simulink model "hoppingControl"  (R2018b)
settings: Solver=FixedStepAuto  StartTime=0.0  StopTime=inf  RelTol=1e-3  EnableMultiTasking=on
libraries: dspstat3 x19, cm_custom x9, raspberrypilib x8, simulink_extras x3, peGeneralControl x3, can_bus_multi x2, simulink x1, embdlinuxlib x1
(part 3 of 3)

== matlab function hoppingControl/Kinematics/MATLAB Function6 ==
  data: theta input; pos output; D input; d input; r input; check output
function [pos, check] = forward_kinematics(theta,D,d,r)
s1 = sin(theta(1)); s2 = sin(theta(2)); s3=sin(theta(3));
c1 = cos(theta(1)); c2 = cos(theta(2)); c3=cos(theta(3));

pos = zeros([3,1]);
knee = zeros([3,3]);
pos(1) =(3^(1/2)*(3*r^3 + D^3*c1*c2^2 + D^3*c2^2*c3 + 2*D*r^2*c1 + 3*D*r^2*c2 + 4*D*r^2*c3 + 2*D^2*r*c2^2 + D^2*r*c1*c2 + 3*D^2*r*c1*c3 + 3*D^2*r*c2*c3 + D^3*c1*c2*c3))/(2*(3*r^2 + D^2*c1*c2 + D^2*c1*c3 + D^2*c2*c3 + 2*D*r*c1 + 2*D*r*c2 + 2*D*r*c3)) - (3^(1/2)*r)/2 - (3^(1/2)*D*c2)/2 + (3^(1/2)*D*(((2*D*s2 + (((c2*s1 + c3*s1 - c2*s3 - c3*s2)*D^2 - r*(s2 - 2*s1 + s3)*D)*(3*r^3 + D^3*c1*c2^2 + D^3*c2^2*c3 + 6*D*r^2*c1 + 3*D*r^2*c2 + 2*D^2*r*c2^2 + 5*D^2*r*c1*c2 + 3*D^2*r*c1*c3 - D^2*r*c2*c3 + D^3*c1*c2*c3))/(3*r^2 + D^2*c1*c2 + D^2*c1*c3 + D^2*c2*c3 + 2*D*r*c1 + 2*D*r*c2 + 2*D*r*c3)^2 - (D*(3*D*sin(theta(1) + theta(2)) - 3*D*sin(theta(1) + theta(3)) + 6*r*s2 - 6*r*s3 - D*sin(theta(1) - theta(2)) + D*sin(theta(1) - theta(3)) + 2*D*sin(theta(2) - theta(3)))*(3*r^3 + D^3*c1*c2^2 + D^3*c2^2*c3 + 2*D*r^2*c1 + 3*D*r^2*c2 + 4*D*r^2*c3 + 2*D^2*r*c2^2 + D^2*r*c1*c2 + 3*D^2*r*c1*c3 + 3*D^2*r*c2*c3 + D^3*c1*c2*c3))/(2*(3*r^2 + D^2*c1*c2 + D^2*c1*c3 + D^2*c2*c3 + 2*D*r*c1 + 2*D*r*c2 + 2*D*r*c3)^2))^2 - ((4*((c2*s1 + c3*s1 - c2*s3 - c3*s2)*D^2 - r*(s2 - 2*s1 + s3)*D)^2)/(3*r^2 + D^2*c1*c2 + D^2*c1*c3 + D^2*c2*c3 + 2*D*r*c1 + 2*D*r*c2 + 2*D*r*c3)^2 + (D^2*(3*D*sin(theta(1) + theta(2)) - 3*D*sin(theta(1) + theta(3)) + 6*r*s2 - 6*r*s3 - D*sin(theta(1) - theta(2)) + D*sin(theta(1) - theta(3)) + 2*D*sin(theta(2) - theta(3)))^2)/(3*(3*r^2 + D^2*c1*c2 + D^2*c1*c3 + D^2*c2*c3 + 2*D*r*c1 + 2*D*r*c2 + 2*D*r*c3)^2) + 4)*((3*r^3 + D^3*c1*c2^2 + D^3*c2^2*c3 + 6*D*r^2*c1 + 3*D*r^2*c2 + 2*D^2*r*c2^2 + 5*D^2*r*c1*c2 + 3*D^2*r*c1*c3 - D^2*r*c2*c3 + D^3*c1*c2*c3)^2/(4*(3*r^2 + D^2*c1*c2 + D^2*c1*c3 + D^2*c2*c3 + 2*D*r*c1 + 2*D*r*c2 + 2*D*r*c3)^2) - D^2*(c2^2 - 1) - d^2 + (3*(3*r^3 + D^3*c1*c2^2 + D^3*c2^2*c3 + 2*D*r^2*c1 + 3*D*r^2*c2 + 4*D*r^2*c3 + 2*D^2*r*c2^2 + D^2*r*c1*c2 + 3*D^2*r*c1*c3 + 3*D^2*r*c2*c3 + D^3*c1*c2*c3)^2)/(4*(3*r^2 + D^2*c1*c2 + D^2*c1*c3 + D^2*c2*c3 + 2*D*r*c1 + 2*D*r*c2 + 2*D*r*c3)^2)))^(1/2)/2 + D*s2 + (((c2*s1 + c3*s1 - c2*s3 - c3*s2)*D^2 - r*(s2 - 2*s1 + s3)*D)*(3*r^3 + D^3*c1*c2^2 + D^3*c2^2*c3 + 6*D*r^2*c1 + 3*D*r^2*c2 + 2*D^2*r*c2^2 + 5*D^2*r*c1*c2 + 3*D^2*r*c1*c3 - D^2*r*c2*c3 + D^3*c1*c2*c3))/(2*(3*r^2 + D^2*c1*c2 + D^2*c1*c3 + D^2*c2*c3 + 2*D*r*c1 + 2*D*r*c2 + 2*D*r*c3)^2) - (D*(3*D*sin(theta(1) + theta(2)) - 3*D*sin(theta(1) + theta(3)) + 6*r*s2 - 6*r*s3 - D*sin(theta(1) - theta(2)) + D*sin(theta(1) - theta(3)) + 2*D*sin(theta(2) - theta(3)))*(3*r^3 + D^3*c1*c2^2 + D^3*c2^2*c3 + 2*D*r^2*c1 + 3*D*r^2*c2 + 4*D*r^2*c3 + 2*D^2*r*c2^2 + D^2*r*c1*c2 + 3*D^2*r*c1*c3 + 3*D^2*r*c2*c3 + D^3*c1*c2*c3))/(4*(3*r^2 + D^2*c1*c2 + D^2*c1*c3 + D^2*c2*c3 + 2*D*r*c1 + 2*D*r*c2 + 2*D*r*c3)^2))*(3*D*sin(theta(1) + theta(2)) - 3*D*sin(theta(1) + theta(3)) + 6*r*s2 - 6*r*s3 - D*sin(theta(1) - theta(2)) + D*sin(theta(1) - theta(3)) + 2*D*sin(theta(2) - theta(3))))/(6*(((c2*s1 + c3*s1 - c2*s3 - c3*s2)*D^2 - r*(s2 - 2*s1 + s3)*D)^2/(3*r^2 + D^2*c1*c2 + D^2*c1*c3 + D^2*c2*c3 + 2*D*r*c1 + 2*D*r*c2 + 2*D*r*c3)^2 + (D^2*(3*D*sin(theta(1) + theta(2)) - 3*D*sin(theta(1) + theta(3)) + 6*r*s2 - 6*r*s3 - D*sin(theta(1) - theta(2)) + D*sin(theta(1) - theta(3)) + 2*D*sin(theta(2) - theta(3)))^2)/(12*(3*r^2 + D^2*c1*c2 + D^2*c1*c3 + D^2*c2*c3 + 2*D*r*c1 + 2*D*r*c2 + 2*D*r*c3)^2) + 1)*(3*r^2 + D^2*c1*c2 + D^2*c1*c3 + D^2*c2*c3 + 2*D*r*c1 + 2*D*r*c2 + 2*D*r*c3));
pos(2) = (3*r^3 + D^3*c1*c2^2 + D^3*c2^2*c3 + 6*D*r^2*c1 + 3*D*r^2*c2 + 2*D^2*r*c2^2 + 5*D^2*r*c1*c2 + 3*D^2*r*c1*c3 - D^2*r*c2*c3 + D^3*c1*c2*c3)/(2*(3*r^2 + D^2*c1*c2 + D^2*c1*c3 + D^2*c2*c3 + 2*D*r*c1 + 2*D*r*c2 + 2*D*r*c3)) - r/2 - (D*c2)/2 - (((c2*s1 + c3*s1 - c2*s3 - c3*s2)*D^2 - r*(s2 - 2*s1 + s3)*D)*(((2*D*s2 + (((c2*s1 + c3*s1 - c2*s3 - c3*s2)*D^2 - r*(s2 - 2*s1 + s3)*D)*(3*r^3 + D^3*c1*c2^2 + D^3*c2^2*c3 + 6*D*r^2*c1 + 3*D*r^2*c2 + 2*D^2*r*c2^2 + 5*D^2*r*c1*c2 + 3*D^2*r*c1*c3 - D^2*r*c2*c3 + D^3*c1*c2*c3))/(3*r^2 + D^2*c1*c2 + D^2*c1*c3 + D^2*c2*c3 + 2*D*r*c1 + 2*D*r*c2 + 2*D*r*c3)^2 - (D*(3*D*sin(theta(1) + theta(2)) - 3*D*sin(theta(1) + theta(3)) + 6*r*s2 - 6*r*s3 - D*sin(theta(1) - theta(2)) + D*sin(theta(1) - theta(3)) + 2*D*sin(theta(2) - theta(3)))*(3*r^3 + D^3*c1*c2^2 + D^3*c2^2*c3 + 2*D*r^2*c1 + 3*D*r^2*c2 + 4*D*r^2*c3 + 2*D^2*r*c2^2 + D^2*r*c1*c2 + 3*D^2*r*c1*c3 + 3*D^2*r*c2*c3 + D^3*c1*c2*c3))/(2*(3*r^2 + D^2*c1*c2 + D^2*c1*c3 + D^2*c2*c3 + 2*D*r*c1 + 2*D*r*c2 + 2*D*r*c3)^2))^2 - ((4*((c2*s1 + c3*s1 - c2*s3 - c3*s2)*D^2 - r*(s2 - 2*s1 + s3)*D)^2)/(3*r^2 + D^2*c1*c2 + D^2*c1*c3 + D^2*c2*c3 + 2*D*r*c1 + 2*D*r*c2 + 2*D*r*c3)^2 + (D^2*(3*D*sin(theta(1) + theta(2)) - 3*D*sin(theta(1) + theta(3)) + 6*r*s2 - 6*r*s3 - D*sin(theta(1) - theta(2)) + D*sin(theta(1) - theta(3)) + 2*D*sin(theta(2) - theta(3)))^2)/(3*(3*r^2 + D^2*c1*c2 + D^2*c1*c3 + D^2*c2*c3 + 2*D*r*c1 + 2*D*r*c2 + 2*D*r*c3)^2) + 4)*((3*r^3 + D^3*c1*c2^2 + D^3*c2^2*c3 + 6*D*r^2*c1 + 3*D*r^2*c2 + 2*D^2*r*c2^2 + 5*D^2*r*c1*c2 + 3*D^2*r*c1*c3 - D^2*r*c2*c3 + D^3*c1*c2*c3)^2/(4*(3*r^2 + D^2*c1*c2 + D^2*c1*c3 + D^2*c2*c3 + 2*D*r*c1 + 2*D*r*c2 + 2*D*r*c3)^2) - D^2*(c2^2 - 1) - d^2 + (3*(3*r^3 + D^3*c1*c2^2 + D^3*c2^2*c3 + 2*D*r^2*c1 + 3*D*r^2*c2 + 4*D*r^2*c3 + 2*D^2*r*c2^2 + D^2*r*c1*c2 + 3*D^2*r*c1*c3 + 3*D^2*r*c2*c3 + D^3*c1*c2*c3)^2)/(4*(3*r^2 + D^2*c1*c2 + D^2*c1*c3 + D^2*c2*c3 + 2*D*r*c1 + 2*D*r*c2 + 2*D*r*c3)^2)))^(1/2)/2 + D*s2 + (((c2*s1 + c3*s1 - c2*s3 - c3*s2)*D^2 - r*(s2 - 2*s1 + s3)*D)*(3*r^3 + D^3*c1*c2^2 + D^3*c2^2*c3 + 6*D*r^2*c1 + 3*D*r^2*c2 + 2*D^2*r*c2^2 + 5*D^2*r*c1*c2 + 3*D^2*r*c1*c3 - D^2*r*c2*c3 + D^3*c1*c2*c3))/(2*(3*r^2 + D^2*c1*c2 + D^2*c1*c3 + D^2*c2*c3 + 2*D*r*c1 + 2*D*r*c2 + 2*D*r*c3)^2) - (D*(3*D*sin(theta(1) + theta(2)) - 3*D*sin(theta(1) + theta(3)) + 6*r*s2 - 6*r*s3 - D*sin(theta(1) - theta(2)) + D*sin(theta(1) - theta(3)) + 2*D*sin(theta(2) - theta(3)))*(3*r^3 + D^3*c1*c2^2 + D^3*c2^2*c3 + 2*D*r^2*c1 + 3*D*r^2*c2 + 4*D*r^2*c3 + 2*D^2*r*c2^2 + D^2*r*c1*c2 + 3*D^2*r*c1*c3 + 3*D^2*r*c2*c3 + D^3*c1*c2*c3))/(4*(3*r^2 + D^2*c1*c2 + D^2*c1*c3 + D^2*c2*c3 + 2*D*r*c1 + 2*D*r*c2 + 2*D*r*c3)^2)))/((((c2*s1 + c3*s1 - c2*s3 - c3*s2)*D^2 - r*(s2 - 2*s1 + s3)*D)^2/(3*r^2 + D^2*c1*c2 + D^2*c1*c3 + D^2*c2*c3 + 2*D*r*c1 + 2*D*r*c2 + 2*D*r*c3)^2 + (D^2*(3*D*sin(theta(1) + theta(2)) - 3*D*sin(theta(1) + theta(3)) + 6*r*s2 - 6*r*s3 - D*sin(theta(1) - theta(2)) + D*sin(theta(1) - theta(3)) + 2*D*sin(theta(2) - theta(3)))^2)/(12*(3*r^2 + D^2*c1*c2 + D^2*c1*c3 + D^2*c2*c3 + 2*D*r*c1 + 2*D*r*c2 + 2*D*r*c3)^2) + 1)*(3*r^2 + D^2*c1*c2 + D^2*c1*c3 + D^2*c2*c3 + 2*D*r*c1 + 2*D*r*c2 + 2*D*r*c3));
pos(3) = (((2*D*s2 + (((c2*s1 + c3*s1 - c2*s3 - c3*s2)*D^2 - r*(s2 - 2*s1 + s3)*D)*(3*r^3 + D^3*c1*c2^2 + D^3*c2^2*c3 + 6*D*r^2*c1 + 3*D*r^2*c2 + 2*D^2*r*c2^2 + 5*D^2*r*c1*c2 + 3*D^2*r*c1*c3 - D^2*r*c2*c3 + D^3*c1*c2*c3))/(3*r^2 + D^2*c1*c2 + D^2*c1*c3 + D^2*c2*c3 + 2*D*r*c1 + 2*D*r*c2 + 2*D*r*c3)^2 - (D*(3*D*sin(theta(1) + theta(2)) - 3*D*sin(theta(1) + theta(3)) + 6*r*s2 - 6*r*s3 - D*sin(theta(1) - theta(2)) + D*sin(theta(1) - theta(3)) + 2*D*sin(theta(2) - theta(3)))*(3*r^3 + D^3*c1*c2^2 + D^3*c2^2*c3 + 2*D*r^2*c1 + 3*D*r^2*c2 + 4*D*r^2*c3 + 2*D^2*r*c2^2 + D^2*r*c1*c2 + 3*D^2*r*c1*c3 + 3*D^2*r*c2*c3 + D^3*c1*c2*c3))/(2*(3*r^2 + D^2*c1*c2 + D^2*c1*c3 + D^2*c2*c3 + 2*D*r*c1 + 2*D*r*c2 + 2*D*r*c3)^2))^2 - ((4*((c2*s1 + c3*s1 - c2*s3 - c3*s2)*D^2 - r*(s2 - 2*s1 + s3)*D)^2)/(3*r^2 + D^2*c1*c2 + D^2*c1*c3 + D^2*c2*c3 + 2*D*r*c1 + 2*D*r*c2 + 2*D*r*c3)^2 + (D^2*(3*D*sin(theta(1) + theta(2)) - 3*D*sin(theta(1) + theta(3)) + 6*r*s2 - 6*r*s3 - D*sin(theta(1) - theta(2)) + D*sin(theta(1) - theta(3)) + 2*D*sin(theta(2) - theta(3)))^2)/(3*(3*r^2 + D^2*c1*c2 + D^2*c1*c3 + D^2*c2*c3 + 2*D*r*c1 + 2*D*r*c2 + 2*D*r*c3)^2) + 4)*((3*r^3 + D^3*c1*c2^2 + D^3*c2^2*c3 + 6*D*r^2*c1 + 3*D*r^2*c2 + 2*D^2*r*c2^2 + 5*D^2*r*c1*c2 + 3*D^2*r*c1*c3 - D^2*r*c2*c3 + D^3*c1*c2*c3)^2/(4*(3*r^2 + D^2*c1*c2 + D^2*c1*c3 + D^2*c2*c3 + 2*D*r*c1 + 2*D*r*c2 + 2*D*r*c3)^2) - D^2*(c2^2 - 1) - d^2 + (3*(3*r^3 + D^3*c1*c2^2 + D^3*c2^2*c3 + 2*D*r^2*c1 + 3*D*r^2*c2 + 4*D*r^2*c3 + 2*D^2*r*c2^2 + D^2*r*c1*c2 + 3*D^2*r*c1*c3 + 3*D^2*r*c2*c3 + D^3*c1*c2*c3)^2)/(4*(3*r^2 + D^2*c1*c2 + D^2*c1*c3 + D^2*c2*c3 + 2*D*r*c1 + 2*D*r*c2 + 2*D*r*c3)^2)))^(1/2)/2 + D*s2 + (((c2*s1 + c3*s1 - c2*s3 - c3*s2)*D^2 - r*(s2 - 2*s1 + s3)*D)*(3*r^3 + D^3*c1*c2^2 + D^3*c2^2*c3 + 6*D*r^2*c1 + 3*D*r^2*c2 + 2*D^2*r*c2^2 + 5*D^2*r*c1*c2 + 3*D^2*r*c1*c3 - D^2*r*c2*c3 + D^3*c1*c2*c3))/(2*(3*r^2 + D^2*c1*c2 + D^2*c1*c3 + D^2*c2*c3 + 2*D*r*c1 + 2*D*r*c2 + 2*D*r*c3)^2) - (D*(3*D*sin(theta(1) + theta(2)) - 3*D*sin(theta(1) + theta(3)) + 6*r*s2 - 6*r*s3 - D*sin(theta(1) - theta(2)) + D*sin(theta(1) - theta(3)) + 2*D*sin(theta(2) - theta(3)))*(3*r^3 + D^3*c1*c2^2 + D^3*c2^2*c3 + 2*D*r^2*c1 + 3*D*r^2*c2 + 4*D*r^2*c3 + 2*D^2*r*c2^2 + D^2*r*c1*c2 + 3*D^2*r*c1*c3 + 3*D^2*r*c2*c3 + D^3*c1*c2*c3))/(4*(3*r^2 + D^2*c1*c2 + D^2*c1*c3 + D^2*c2*c3 + 2*D*r*c1 + 2*D*r*c2 + 2*D*r*c3)^2))/(((c2*s1 + c3*s1 - c2*s3 - c3*s2)*D^2 - r*(s2 - 2*s1 + s3)*D)^2/(3*r^2 + D^2*c1*c2 + D^2*c1*c3 + D^2*c2*c3 + 2*D*r*c1 + 2*D*r*c2 + 2*D*r*c3)^2 + (D^2*(3*D*sin(theta(1) + theta(2)) - 3*D*sin(theta(1) + theta(3)) + 6*r*s2 - 6*r*s3 - D*sin(theta(1) - theta(2)) + D*sin(theta(1) - theta(3)) + 2*D*sin(theta(2) - theta(3)))^2)/(12*(3*r^2 + D^2*c1*c2 + D^2*c1*c3 + D^2*c2*c3 + 2*D*r*c1 + 2*D*r*c2 + 2*D*r*c3)^2) + 1);
for i = 1:3
    R =  [cosd(120*(i-1)) -sind(120*(i-1)) 0; sind(120*(i-1)) cosd(120*(i-1)) 0; 0 0 1];
    knee(:,i) = R*([0;17.75;0]+[0;D*cos(theta(i));D*sin(theta(i))]);
end

for i = 1:3
    R =  [cosd(120*(i-1)) -sind(120*(i-1)) 0; sind(120*(i-1)) cosd(120*(i-1)) 0; 0 0 1];
    knee(:,i) = R*([0;r;0]+[0;D*cos(theta(i));D*sin(theta(i))]);
end
check = zeros([3,1]);
check(1) = dot(pos-knee(:,1),pos-knee(:,1))-d^2;
check(2) = dot(pos-knee(:,2),pos-knee(:,2))-d^2;
check(3) = dot(pos-knee(:,3),pos-knee(:,3))-d^2;
end

== matlab function hoppingControl/Kinematics/MATLAB Function7 ==
  data: x input; thetadot input; j output; D input; d input; r input; xdot output
function [j,xdot] = inverse_jacobian(x,thetadot,D,d,r)

j = [                                                                                                                                                                                                                                                                                                                                                                                                x(1)/(D*((r - x(2))^2 + x(3)^2)^(1/2)*(1 - ((r - x(2))^2/2 + D^2/2 - d^2/2 + x(1)^2/2 + x(3)^2/2)^2/(D^2*((r - x(2))^2 + x(3)^2)))^(1/2)),                                                                                                                                                                                                                                           - ((r - x(2))/(D*((r - x(2))^2 + x(3)^2)^(1/2)) - ((2*r - 2*x(2))*((r - x(2))^2/2 + D^2/2 - d^2/2 + x(1)^2/2 + x(3)^2/2))/(2*D*((r - x(2))^2 + x(3)^2)^(3/2)))/(1 - ((r - x(2))^2/2 + D^2/2 - d^2/2 + x(1)^2/2 + x(3)^2/2)^2/(D^2*((r - x(2))^2 + x(3)^2)))^(1/2) - x(3)/((r - x(2))^2 + x(3)^2),                                                                                                  (x(3)/(D*((r - x(2))^2 + x(3)^2)^(1/2)) - (x(3)*((r - x(2))^2/2 + D^2/2 - d^2/2 + x(1)^2/2 + x(3)^2/2))/(D*((r - x(2))^2 + x(3)^2)^(3/2)))/(1 - ((r - x(2))^2/2 + D^2/2 - d^2/2 + x(1)^2/2 + x(3)^2/2)^2/(D^2*((r - x(2))^2 + x(3)^2)))^(1/2) - (r - x(2))/((r - x(2))^2 + x(3)^2);
 ((x(1)/4 - (3^(1/2)*x(2))/4 + (3^(1/2)*(r + x(2)/2 + (3^(1/2)*x(1))/2))/2)/(D*((r + x(2)/2 + (3^(1/2)*x(1))/2)^2 + x(3)^2)^(1/2)) - (3^(1/2)*(r + x(2)/2 + (3^(1/2)*x(1))/2)*((r + x(2)/2 + (3^(1/2)*x(1))/2)^2/2 + D^2/2 - d^2/2 + (x(1)/2 - (3^(1/2)*x(2))/2)^2/2 + x(3)^2/2))/(2*D*((r + x(2)/2 + (3^(1/2)*x(1))/2)^2 + x(3)^2)^(3/2)))/(- ((r + x(2)/2 + (3^(1/2)*x(1))/2)^2/2 + D^2/2 - d^2/2 + (x(1)/2 - (3^(1/2)*x(2))/2)^2/2 + x(3)^2/2)^2/(D^2*((r + x(2)/2 + (3^(1/2)*x(1))/2)^2 + x(3)^2)) + 1)^(1/2) + (3^(1/2)*x(3))/(2*((r + x(2)/2 + (3^(1/2)*x(1))/2)^2 + x(3)^2)), x(3)/(2*((r + x(2)/2 + (3^(1/2)*x(1))/2)^2 + x(3)^2)) + ((r/2 + x(2)/4 - (3^(1/2)*(x(1)/2 - (3^(1/2)*x(2))/2))/2 + (3^(1/2)*x(1))/4)/(D*((r + x(2)/2 + (3^(1/2)*x(1))/2)^2 + x(3)^2)^(1/2)) - ((r + x(2)/2 + (3^(1/2)*x(1))/2)*((r + x(2)/2 + (3^(1/2)*x(1))/2)^2/2 + D^2/2 - d^2/2 + (x(1)/2 - (3^(1/2)*x(2))/2)^2/2 + x(3)^2/2))/(2*D*((r + x(2)/2 + (3^(1/2)*x(1))/2)^2 + x(3)^2)^(3/2)))/(- ((r + x(2)/2 + (3^(1/2)*x(1))/2)^2/2 + D^2/2 - d^2/2 + (x(1)/2 - (3^(1/2)*x(2))/2)^2/2 + x(3)^2/2)^2/(D^2*((r + x(2)/2 + (3^(1/2)*x(1))/2)^2 + x(3)^2)) + 1)^(1/2), (2*x(3)*(- 2*D^2 + 2*d^2 + 2*r^2 + 2*3^(1/2)*r*x(1) + 2*r*x(2) + x(1)^2 + 2*3^(1/2)*x(1)*x(2) - x(2)^2 + 2*x(3)^2))/(D*(- (r*x(2) + D^2 - d^2 + r^2 + x(1)^2 + x(2)^2 + x(3)^2 + 3^(1/2)*r*x(1))^2/(D^2*((2*r + x(2) + 3^(1/2)*x(1))^2 + 4*x(3)^2)) + 1)^(1/2)*((2*r + x(2) + 3^(1/2)*x(1))^2 + 4*x(3)^2)^(3/2)) - (4*(r + x(2)/2 + (3^(1/2)*x(1))/2))/((2*r + x(2) + 3^(1/2)*x(1))^2 + 4*x(3)^2);
 ((x(1)/4 + (3^(1/2)*x(2))/4 - (3^(1/2)*(r + x(2)/2 - (3^(1/2)*x(1))/2))/2)/(D*((r + x(2)/2 - (3^(1/2)*x(1))/2)^2 + x(3)^2)^(1/2)) + (3^(1/2)*(r + x(2)/2 - (3^(1/2)*x(1))/2)*((r + x(2)/2 - (3^(1/2)*x(1))/2)^2/2 + D^2/2 - d^2/2 + (x(1)/2 + (3^(1/2)*x(2))/2)^2/2 + x(3)^2/2))/(2*D*((r + x(2)/2 - (3^(1/2)*x(1))/2)^2 + x(3)^2)^(3/2)))/(- ((r + x(2)/2 - (3^(1/2)*x(1))/2)^2/2 + D^2/2 - d^2/2 + (x(1)/2 + (3^(1/2)*x(2))/2)^2/2 + x(3)^2/2)^2/(D^2*((r + x(2)/2 - (3^(1/2)*x(1))/2)^2 + x(3)^2)) + 1)^(1/2) - (3^(1/2)*x(3))/(2*((r + x(2)/2 - (3^(1/2)*x(1))/2)^2 + x(3)^2)), x(3)/(2*((r + x(2)/2 - (3^(1/2)*x(1))/2)^2 + x(3)^2)) + ((r/2 + x(2)/4 + (3^(1/2)*(x(1)/2 + (3^(1/2)*x(2))/2))/2 - (3^(1/2)*x(1))/4)/(D*((r + x(2)/2 - (3^(1/2)*x(1))/2)^2 + x(3)^2)^(1/2)) - ((r + x(2)/2 - (3^(1/2)*x(1))/2)*((r + x(2)/2 - (3^(1/2)*x(1))/2)^2/2 + D^2/2 - d^2/2 + (x(1)/2 + (3^(1/2)*x(2))/2)^2/2 + x(3)^2/2))/(2*D*((r + x(2)/2 - (3^(1/2)*x(1))/2)^2 + x(3)^2)^(3/2)))/(- ((r + x(2)/2 - (3^(1/2)*x(1))/2)^2/2 + D^2/2 - d^2/2 + (x(1)/2 + (3^(1/2)*x(2))/2)^2/2 + x(3)^2/2)^2/(D^2*((r + x(2)/2 - (3^(1/2)*x(1))/2)^2 + x(3)^2)) + 1)^(1/2), (2*x(3)*(- 2*D^2 + 2*d^2 + 2*r^2 - 2*3^(1/2)*r*x(1) + 2*r*x(2) + x(1)^2 - 2*3^(1/2)*x(1)*x(2) - x(2)^2 + 2*x(3)^2))/(D*(- (r*x(2) + D^2 - d^2 + r^2 + x(1)^2 + x(2)^2 + x(3)^2 - 3^(1/2)*r*x(1))^2/(D^2*((2*r + x(2) - 3^(1/2)*x(1))^2 + 4*x(3)^2)) + 1)^(1/2)*((2*r + x(2) - 3^(1/2)*x(1))^2 + 4*x(3)^2)^(3/2)) - (4*(r + x(2)/2 - (3^(1/2)*x(1))/2))/((2*r + x(2) - 3^(1/2)*x(1))^2 + 4*x(3)^2)];
xdot = j\thetadot(1:3);


end

== stateflow chart hoppingControl/state estimation/Chart ==
  state imu_init
    entry:
    state enableWrite
      entry:
      imu_err = enable_write();
    state parsing
    state enableData
      entry:
      imu_err = enable_data();
    state parsing1
    state setFrequency
      entry:
      imu_err = set_freq();
    state parsing2
    state setAccelRange
      entry:
      imu_err = set_accel();
    state parsing3
    state setGyroRange
      entry:
      imu_err = set_gyro();
    state parsing4
    state setFilterMode
      entry:
      imu_err = set_filter();
    state parsing5
    state disableWrite
      entry:
      imu_err = disable_write();
    (default) -> enableWrite
    enableWrite -> parsing : [imu_err == 0]
    parsing -> enableData : after(0.1,sec)
    enableData -> parsing1 : [imu_err == 0]
    parsing1 -> setFrequency : after(0.1,sec)
    setFrequency -> parsing2 : [imu_err == 0]
    parsing2 -> setAccelRange : after(0.1,sec)
    setAccelRange -> parsing3 : [imu_err == 0]
    parsing3 -> setGyroRange : after(0.1,sec)
    setGyroRange -> parsing4 : [imu_err == 0]
    parsing4 -> setFilterMode : after(0.1,sec)
    setFilterMode -> parsing5 : [imu_err == 0]
    parsing5 -> disableWrite : after(0.1,sec)
  state imu_read
    during:
    state badRead
    state readData
      entry:
      acc = raw_acc;
      gyro = raw_gyro;
    (junction 72) -> (junction 73) : {[raw_acc,raw_gyro,imu_err] = read_imu();}
    (junction 73) -> badRead [order 2]
    badRead -> (junction 72)
    readData -> (junction 72)
    (junction 73) -> readData [order 1] : [imu_err == 0]
  state [acc,gyro,err] = read_imu [function]
  state err = enable_write [function]
  state err = enable_data [function]
  state err = set_freq [function]
  state err = set_accel [function]
  state err = set_gyro [function]
  state err = set_filter [function]
  state err = disable_write [function]
  (default) -> imu_init
  (junction 56) -> (junction 72)
  (junction 57) -> (junction 56)
  disableWrite -> (junction 57) : after(0.1,sec)
  data: acc function_output; gyro function_output; err function_output; err function_output; err function_output; err function_output; err function_output; err function_output; err function_output; err function_output; acc output; gyro output; raw_gyro local; raw_acc local; imu_err local
